simulink model "BLDC_model"  (R2021a)
settings: Solver=ode23t  StartTime=0.0  StopTime=3  RelTol=1e-3
libraries: spsMosfetLib x6, spsVoltageMeasurementLib x3, spsControlledVoltageSourceLib x1, spspowerguiLib x1
settings Model: Creator=Deepak  LastModifiedBy=Hossam
settings SolverCC: AlgebraicLoopSolver=TrustRegion
settings OptimizationCC: UseDivisionForNetSlopeComputation=on
settings DebuggingCC: SFMachineParentedDataDiag=warning
settings SFSimCC: CustomCodeUndefinedFunction=UseInterfaceOnly

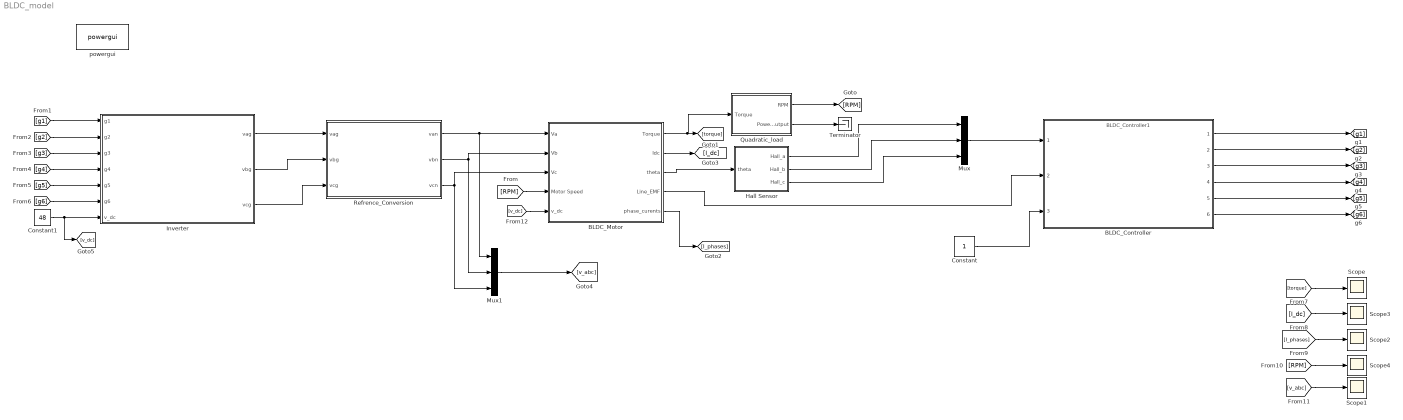
== system BLDC_model ==
  BLDC_Controller : ModelReference  ModelNameDialog=BLDC_Controller1  SimulationMode=Software-in-the-loop (SIL)  ModelReferenceVersion=2.12
  BLDC_Motor : Subsystem
  Constant : Constant  OutDataTypeStr=boolean
  Constant1 : Constant  Value=48
  Hall Sensor : Subsystem
  Inverter : Subsystem
  Mux : Mux  Inputs=3
  Mux1 : Mux  Inputs=3
  Quadratic_load : Subsystem
  Refrence_Conversion : Subsystem
  Scope{,1..4} (5 alike) : Scope
  Terminator : Terminator
  powergui : spspowerguiLib/powergui  Priority=1  SimulationMode=Discrete  SampleTime=50e-6  frequency=60  Iterations=50  frequencyindice=0  Pbase=100e6  ErrMax=1e-4  UnitsV=kV  UnitsW=MW  buscounter=0  FunctionMessages=off  echomessages=off  EnableUseOfTLC=off  CurrentSourceSwitches=off  DisableSnubberDevices=off  DisableRonSwitches=off  DisableVfSwitches=off  DisplayEquations=off  AutomaticDiscreteSolvers=off  SolverType=Tustin/Backward Euler (TBE)  Interpol=off  ExternalGateDelay=off  methode=off  Ts=100  x0status=blocks  SPID=on  SwTol=0  HookPort=off  NonlinearTolerance=0  nMaxIteration=15  ContinueOnMaxIteration=off  RestoreLinks=warning  ResistiveCurrentMeasurement=off  Frange=[0:2:500]  Ylog=off  Xlog=on  ShowGrid=off  save=off  variable=ZData  structure=0  ZoomFFT=off  StartTime=0.0  cycles=1  DisplayStyle=1  fundamental=60  FreqAxis=off  MaxFrequency=1000  frequencyindicesteady=1  RmsSteady=1  display=off
  wires:
  BLDC_Motor/3(theta) -> Hall Sensor/1(theta)
  Hall Sensor/1(Hall_a) -> Mux/1
  Hall Sensor/2(Hall_b) -> Mux/2
  Hall Sensor/3(Hall_c) -> Mux/3
  BLDC_Motor/1(Torque) -> Quadratic_load/1(Torque), [torque]
  Refrence_Conversion/2(vbn) -> Mux1/2, BLDC_Motor/2(Vb)
  Refrence_Conversion/3(vcn) -> BLDC_Motor/3(Vc), Mux1/3
  [RPM] -> BLDC_Motor/4(Motor Speed)
  Quadratic_load/1(RPM) -> [RPM]
  BLDC_Controller/1 -> [g1]
  BLDC_Controller/2 -> [g2]
  BLDC_Controller/3 -> [g3]
  BLDC_Controller/4 -> [g4]
  BLDC_Controller/5 -> [g5]
  BLDC_Controller/6 -> [g6]
  [g1] -> Inverter/1(g1)
  [g2] -> Inverter/2(g2)
  [g3] -> Inverter/3(g3)
  [g4] -> Inverter/4(g4)
  [g5] -> Inverter/5(g5)
  [g6] -> Inverter/6(g6)
  Inverter/3(vcg) -> Refrence_Conversion/3(vcg)
  Inverter/2(vbg) -> Refrence_Conversion/2(vbg)
  Inverter/1(vag) -> Refrence_Conversion/1(vag)
  Mux/1 -> BLDC_Controller/1
  Quadratic_load/2(PowerOutput) -> Terminator/1
  BLDC_Motor/2(Idc) -> [I_dc]
  Constant/1 -> BLDC_Controller/3
  BLDC_Motor/4(Line_EMF) -> BLDC_Controller/2
  [torque] -> Scope/1
  BLDC_Motor/5(phase_curents) -> [I_phases]
  [I_dc] -> Scope3/1
  [I_phases] -> Scope2/1
  [RPM] -> Scope4/1
  Mux1/1 -> [v_abc]
  [v_abc] -> Scope1/1
  Refrence_Conversion/1(van) -> Mux1/1, BLDC_Motor/1(Va)
  Constant1/1 -> [v_dc], Inverter/7(v_dc)
  [v_dc] -> BLDC_Motor/5(v_dc)

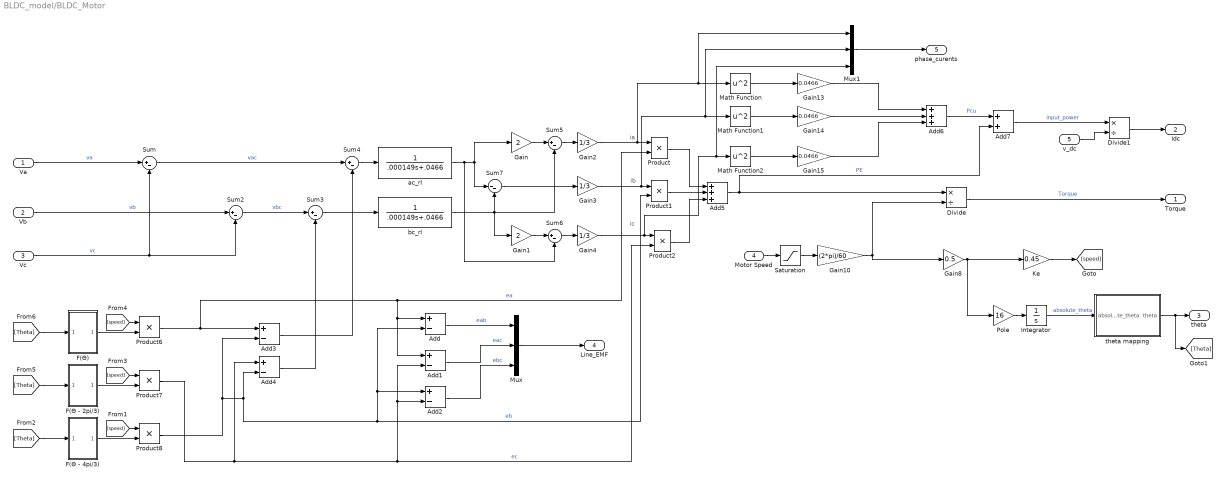
== system BLDC_model/BLDC_Motor ==
  note: ic
  note: ib
  note: ia
  Va : Inport
  Vb : Inport  Port=2
  Vc : Inport  Port=3
  Motor Speed : Inport  Port=4
  v_dc : Inport  Port=5
  Add{,2..4} (4 alike) : Sum  Inputs=+-
  Add1 : Sum  Inputs=+-  AccumDataTypeStr=double
  Add5 : Sum  Inputs=+++
  Add6 : Sum  Inputs=+++
  Add7 : Sum
  Divide : Product  Inputs=*/
  Divide1 : Product  Inputs=*/
  F(Θ - 2pi/3) : Subsystem
  F(Θ - 4pi/3) : Subsystem
  F(Θ) : Subsystem
  Gain : Gain  Gain=2
  Gain1 : Gain  Gain=2
  Gain10 : Gain  Gain=(2*pi)/60
  Gain13 : Gain  Gain=0.0466
  Gain14 : Gain  Gain=0.0466
  Gain15 : Gain  Gain=0.0466
  Gain2 : Gain  Gain=1/3
  Gain3 : Gain  Gain=1/3
  Gain4 : Gain  Gain=1/3
  Gain8 : Gain  Gain=0.5
  Integrator : Integrator
  Ke : Gain  Gain=0.45
  Math Function : Math  Operator=square  SaturateOnIntegerOverflow=on
  Math Function1 : Math  Operator=square  SaturateOnIntegerOverflow=on
  Math Function2 : Math  Operator=square  SaturateOnIntegerOverflow=on
  Mux : Mux  Inputs=3
  Mux1 : Mux  Inputs=3
  Pole : Gain  Gain=16
  Product{,1..2,6..8} (6 alike) : Product
  Saturation : Saturate  UpperLimit=50000  LowerLimit=1
  Sum{,2..6} (6 alike) : Sum  Inputs=|+-
  Sum7 : Sum  Inputs=|--
  ac_rl : TransferFcn  Denominator=[.000149 .0466]
  bc_rl : TransferFcn  Denominator=[.000149 .0466]
  theta mapping : Subsystem
  Torque : Outport
  Idc : Outport  Port=2
  theta : Outport  Port=3
  Line_EMF : Outport  Port=4
  phase_curents : Outport  Port=5
  wires:
  Pole/1 -> Integrator/1
  Sum7/1 -> Gain3/1
  Sum4/1 -> ac_rl/1
  Sum6/1 -> Gain4/1
  Add4/1 -> Sum3/2
  Vc/1 -> Sum2/2, Sum/2  "vc"
  Gain4/1 -> Mux1/3, Math Function2/1, Product2/1
  Gain2/1 -> Mux1/1, Math Function/1, Product/1
  Gain/1 -> Sum5/1
  Sum3/1 -> bc_rl/1
  Add5/1 -> Add7/2, Divide/1  "PE"
  Vb/1 -> Sum2/1  "vb"
  Sum/1 -> Sum4/1  "vac"
  bc_rl/1 -> Gain1/1, Sum5/2, Sum7/2
  Gain8/1 -> Ke/1, Pole/1
  Gain1/1 -> Sum6/1
  Product/1 -> Add5/1
  Gain3/1 -> Mux1/2, Math Function1/1, Product1/1
  Add3/1 -> Sum4/2
  Product7/1 -> Add4/1, Product2/2, Add2/2, Add1/2  "ec"
  Sum5/1 -> Gain2/1
  Product2/1 -> Add5/3
  Sum2/1 -> Sum3/1  "vbc"
  Product6/1 -> Add3/1, Add1/1, Add/1, Product/2  "ea"
  Integrator/1 -> theta mapping/1(absolute_theta)  "absolute_theta"
  Product1/1 -> Add5/2
  ac_rl/1 -> Gain/1, Sum7/1, Sum6/2
  Va/1 -> Sum/1  "va"
  Divide/1 -> Torque/1  "Torque"
  Motor Speed/1 -> Saturation/1
  Saturation/1 -> Gain10/1
  Math Function/1 -> Gain13/1
  Math Function1/1 -> Gain14/1
  Math Function2/1 -> Gain15/1
  Gain13/1 -> Add6/1
  Gain14/1 -> Add6/2
  Gain15/1 -> Add6/3
  Add6/1 -> Add7/1  "Pcu"
  Add7/1 -> Divide1/1  "input_power"
  Divide1/1 -> Idc/1
  Add/1 -> Mux/1  "eab"
  Add1/1 -> Mux/2  "eac"
  Add2/1 -> Mux/3  "ebc"
  Mux/1 -> Line_EMF/1
  Gain10/1 -> Divide/2, Gain8/1
  Ke/1 -> [speed]
  theta mapping/1(theta) -> [Theta], theta/1
  F(Θ)/1(Out1) -> Product6/2
  F(Θ - 2pi/3)/1(Out1) -> Product7/2
  F(Θ - 4pi/3)/1(Out1) -> Product8/2
  Product8/1 -> Add3/2, Product1/2, Add/2, Add2/1, Add4/2  "eb"
  [speed] -> Product8/1
  [speed] -> Product7/1
  [speed] -> Product6/1
  [Theta] -> F(Θ - 4pi/3)/1(In1)
  [Theta] -> F(Θ - 2pi/3)/1(In1)
  [Theta] -> F(Θ)/1(In1)
  Mux1/1 -> phase_curents/1
  v_dc/1 -> Divide1/2

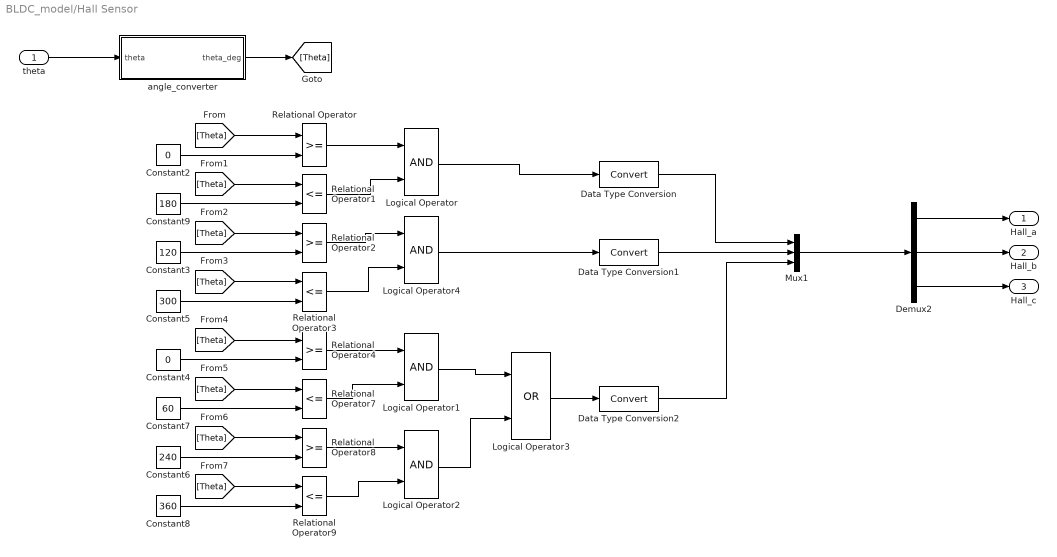
== system BLDC_model/Hall Sensor ==
  theta : Inport
  Constant2 : Constant  Value=0
  Constant3 : Constant  Value=120
  Constant4 : Constant  Value=0
  Constant5 : Constant  Value=300
  Constant6 : Constant  Value=240
  Constant7 : Constant  Value=60
  Constant8 : Constant  Value=360
  Constant9 : Constant  Value=180
  Data Type Conversion : DataTypeConversion
  Data Type Conversion1 : DataTypeConversion
  Data Type Conversion2 : DataTypeConversion
  Demux2 : Demux  Outputs=3
  Logical Operator{,1..2,4} (4 alike) : Logic  AllPortsSameDT=off  OutDataTypeStr=boolean
  Logical Operator3 : Logic  Operator=OR  AllPortsSameDT=off  OutDataTypeStr=boolean
  Mux1 : Mux  Inputs=3
  Relational Operator{,2,4,8} (4 alike) : RelationalOperator  OutDataTypeStr=boolean  RndMeth=Nearest
  Relational Operator{1,3,7,9} (4 alike) : RelationalOperator  Operator=<=  OutDataTypeStr=boolean  RndMeth=Nearest
  angle_converter : Subsystem
  Hall_a : Outport
  Hall_b : Outport  Port=2
  Hall_c : Outport  Port=3
  wires:
  Constant7/1 -> Relational Operator7/2
  Constant3/1 -> Relational Operator2/2
  Relational Operator1/1 -> Logical Operator/2
  Constant9/1 -> Relational Operator1/2
  Relational Operator7/1 -> Logical Operator1/2
  Relational Operator4/1 -> Logical Operator1/1
  Constant2/1 -> Relational Operator/2
  Data Type Conversion/1 -> Mux1/1
  Mux1/1 -> Demux2/1
  Constant4/1 -> Relational Operator4/2
  Relational Operator2/1 -> Logical Operator4/1
  Data Type Conversion1/1 -> Mux1/2
  Constant5/1 -> Relational Operator3/2
  theta/1 -> angle_converter/1(theta)
  Relational Operator/1 -> Logical Operator/1
  Relational Operator3/1 -> Logical Operator4/2
  Logical Operator4/1 -> Data Type Conversion1/1
  Data Type Conversion2/1 -> Mux1/3
  Logical Operator/1 -> Data Type Conversion/1
  Demux2/2 -> Hall_b/1
  Relational Operator8/1 -> Logical Operator2/1
  Relational Operator9/1 -> Logical Operator2/2
  Constant6/1 -> Relational Operator8/2
  Logical Operator1/1 -> Logical Operator3/1
  Logical Operator2/1 -> Logical Operator3/2
  Logical Operator3/1 -> Data Type Conversion2/1
  Demux2/3 -> Hall_c/1
  Demux2/1 -> Hall_a/1
  angle_converter/1(theta_deg) -> [Theta]
  [Theta] -> Relational Operator/1
  [Theta] -> Relational Operator1/1
  [Theta] -> Relational Operator2/1
  [Theta] -> Relational Operator3/1
  [Theta] -> Relational Operator4/1
  [Theta] -> Relational Operator7/1
  [Theta] -> Relational Operator8/1
  Constant8/1 -> Relational Operator9/2
  [Theta] -> Relational Operator9/1

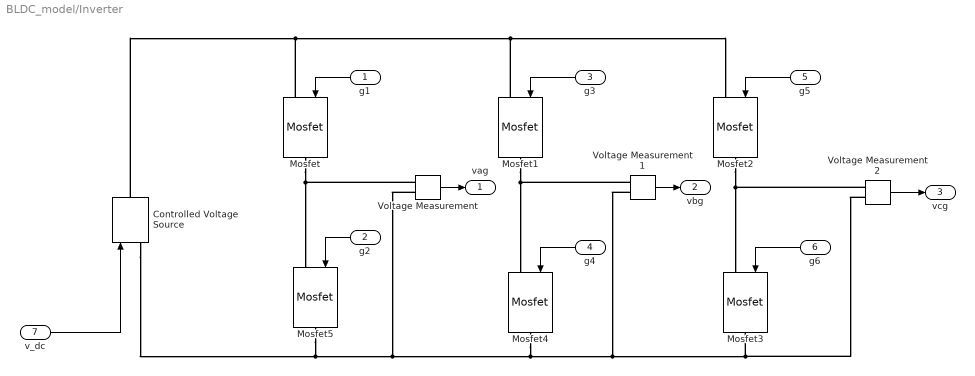
== system BLDC_model/Inverter ==
  g1 : Inport
  g2 : Inport  Port=2
  g3 : Inport  Port=3
  g4 : Inport  Port=4
  g5 : Inport  Port=5
  g6 : Inport  Port=6
  v_dc : Inport  Port=7
  Controlled Voltage Source : spsControlledVoltageSourceLib/Controlled Voltage Source  Initialize=on  Source_Type=DC  Amplitude=48  Phase=0  Frequency=0  Measurements=None
  Mosfet{,1..5} (6 alike) : spsMosfetLib/Mosfet  Ron=0.1  Lon=0  Rd=0.01  Vfd=0  IC=0  Rs=1e5  Cs=inf  Measurements=off
  Voltage Measurement : spsVoltageMeasurementLib/Voltage Measurement  PhasorSimulation=off  OutputType=Complex  PSBequivalent=0
  Voltage Measurement1 : spsVoltageMeasurementLib/Voltage Measurement  PhasorSimulation=off  OutputType=Complex  PSBequivalent=0
  Voltage Measurement2 : spsVoltageMeasurementLib/Voltage Measurement  PhasorSimulation=off  OutputType=Complex  PSBequivalent=0
  vag : Outport
  vbg : Outport  Port=2
  vcg : Outport  Port=3
  wires:
  v_dc/1 -> Controlled Voltage Source/1
  g6/1 -> Mosfet3/1
  g4/1 -> Mosfet4/1
  g3/1 -> Mosfet1/1
  g1/1 -> Mosfet/1
  g5/1 -> Mosfet2/1
  g2/1 -> Mosfet5/1
  Voltage Measurement/1 -> vag/1
  Voltage Measurement1/1 -> vbg/1
  Voltage Measurement2/1 -> vcg/1
  connections:
  Mosfet/LConn1 -- Controlled Voltage Source/RConn1 -- Mosfet1/LConn1 -- Mosfet2/LConn1
  Mosfet2/RConn1 -- Voltage Measurement2/LConn1 -- Mosfet3/LConn1
  Mosfet5/RConn1 -- Mosfet4/RConn1 -- Mosfet3/RConn1 -- Voltage Measurement2/LConn2 -- Voltage Measurement1/LConn2 -- Voltage Measurement/LConn2 -- Controlled Voltage Source/LConn1
  Mosfet1/RConn1 -- Mosfet4/LConn1 -- Voltage Measurement1/LConn1
  Mosfet/RConn1 -- Voltage Measurement/LConn1 -- Mosfet5/LConn1

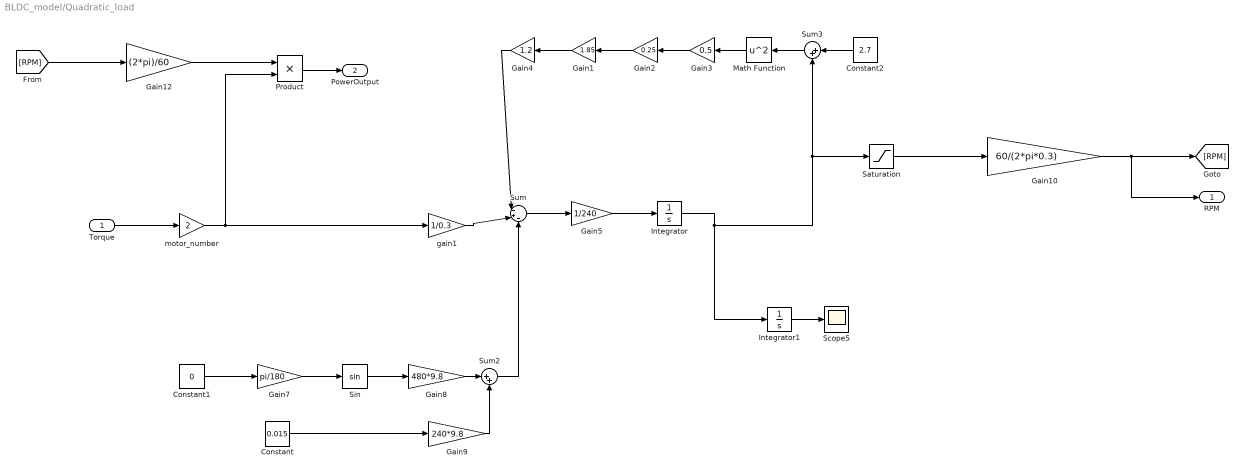
== system BLDC_model/Quadratic_load ==
  Torque : Inport
  Constant : Constant  Value=0.015
  Constant1 : Constant  Value=0
  Constant2 : Constant  Value=2.7
  Gain1 : Gain  Gain=1.85
  Gain10 : Gain  Gain=60/(2*pi*0.3)
  Gain12 : Gain  Gain=(2*pi)/60
  Gain2 : Gain  Gain=0.25
  Gain3 : Gain  Gain=0.5
  Gain4 : Gain  Gain=1.2
  Gain5 : Gain  Gain=1/240
  Gain7 : Gain  Gain=pi/180
  Gain8 : Gain  Gain=480*9.8
  Gain9 : Gain  Gain=240*9.8
  Integrator : Integrator
  Integrator1 : Integrator
  Math Function : Math  Operator=square  SaturateOnIntegerOverflow=on
  Product : Product
  Saturation : Saturate  UpperLimit=50000  LowerLimit=0
  Scope5 : Scope
  Sin : Trigonometry
  Sum : Sum  Inputs=|-+-
  Sum2 : Sum  Inputs=|++
  Sum3 : Sum  Inputs=|++
  gain1 : Gain  Gain=1/0.3
  motor_number : Gain  Gain=2
  RPM : Outport
  PowerOutput : Outport  Port=2
  wires:
  Gain10/1 -> RPM/1, [RPM]
  Sum2/1 -> Sum/3
  Gain7/1 -> Sin/1
  Gain8/1 -> Sum2/1
  Sin/1 -> Gain8/1
  Gain9/1 -> Sum2/2
  Gain2/1 -> Gain1/1
  Gain4/1 -> Sum/1
  gain1/1 -> Sum/2
  Gain1/1 -> Gain4/1
  Sum3/1 -> Math Function/1
  Constant2/1 -> Sum3/1
  Integrator/1 -> Integrator1/1, Saturation/1, Sum3/2
  Product/1 -> PowerOutput/1
  Gain5/1 -> Integrator/1
  Constant1/1 -> Gain7/1
  Constant/1 -> Gain9/1
  Sum/1 -> Gain5/1
  Math Function/1 -> Gain3/1
  Gain3/1 -> Gain2/1
  Torque/1 -> motor_number/1
  Saturation/1 -> Gain10/1
  motor_number/1 -> Product/2, gain1/1
  Integrator1/1 -> Scope5/1
  [RPM] -> Gain12/1
  Gain12/1 -> Product/1

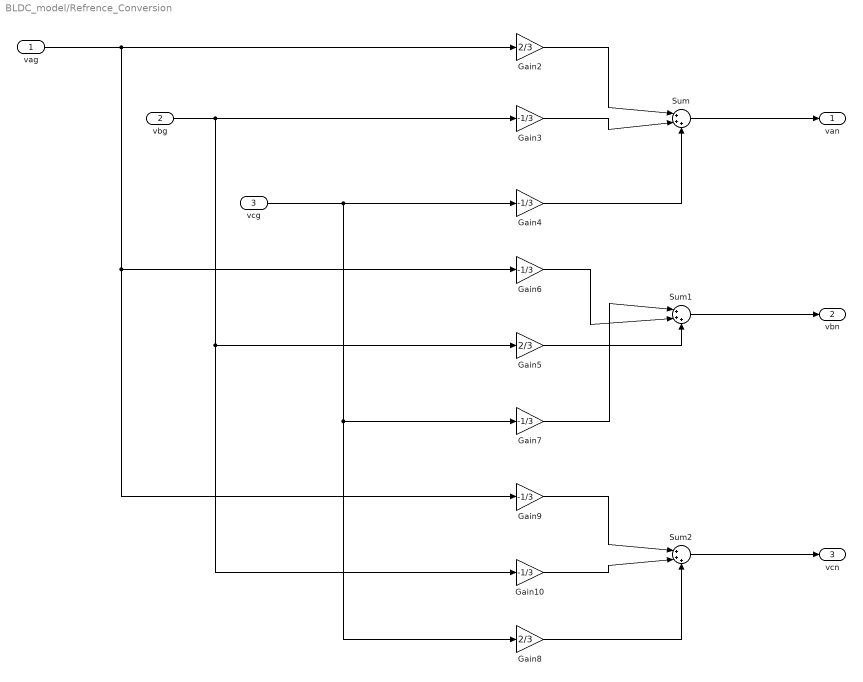
== system BLDC_model/Refrence_Conversion ==
  vag : Inport
  vbg : Inport  Port=2
  vcg : Inport  Port=3
  Gain{3..4,6..7,9..10} (6 alike) : Gain  Gain=-1/3
  Gain2 : Gain  Gain=2/3
  Gain5 : Gain  Gain=2/3
  Gain8 : Gain  Gain=2/3
  Sum : Sum  Inputs=|+++
  Sum1 : Sum  Inputs=|+++
  Sum2 : Sum  Inputs=|+++
  van : Outport
  vbn : Outport  Port=2
  vcn : Outport  Port=3
  wires:
  Gain10/1 -> Sum2/2
  Gain9/1 -> Sum2/1
  Gain8/1 -> Sum2/3
  Gain7/1 -> Sum1/1
  Gain4/1 -> Sum/3
  Gain3/1 -> Sum/2
  vbg/1 -> Gain10/1, Gain5/1, Gain3/1
  Gain6/1 -> Sum1/2
  Gain2/1 -> Sum/1
  vcg/1 -> Gain8/1, Gain7/1, Gain4/1
  Gain5/1 -> Sum1/3
  vag/1 -> Gain2/1, Gain6/1, Gain9/1
  Sum/1 -> van/1
  Sum1/1 -> vbn/1
  Sum2/1 -> vcn/1

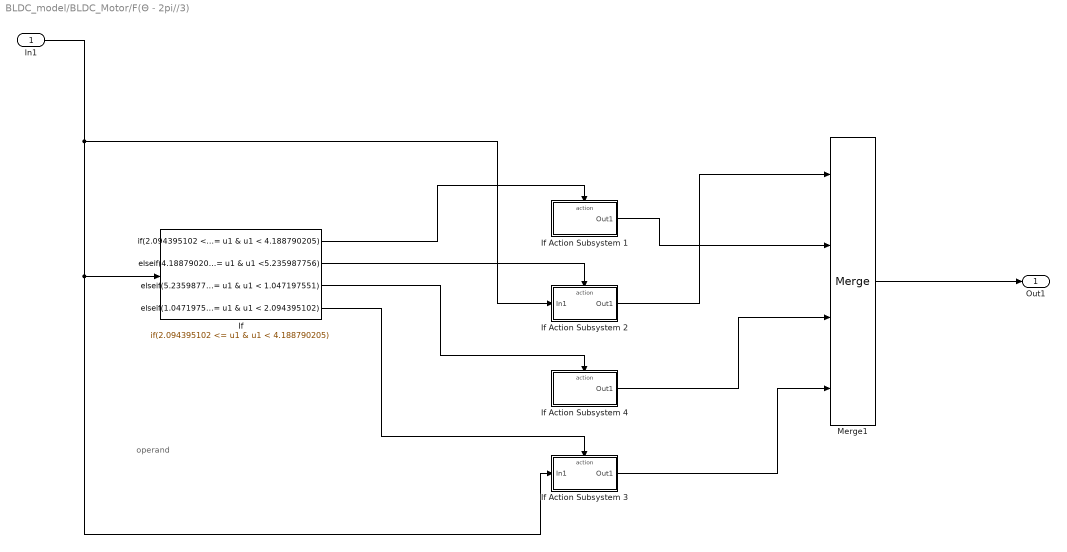
== system BLDC_model/BLDC_Motor/F(Θ - 2pi//3) ==
  note: operand
  In1 : Inport
  If : If  IfExpression=2.094395102 <= u1 & u1 < 4.188790205  ElseIfExpressions=4.188790205 <= u1 & u1 <5.235987756 , 5.235987756>= u1 & u1 < 1.047197551 , 1.047197551 <= u1 & u1 < 2.094395102  ShowElse=off
  If Action Subsystem 1 : Subsystem  TreatAsAtomicUnit=on
  If Action Subsystem 2 : Subsystem  TreatAsAtomicUnit=on
  If Action Subsystem 3 : Subsystem  TreatAsAtomicUnit=on
  If Action Subsystem 4 : Subsystem  TreatAsAtomicUnit=on
  Merge1 : Merge  Inputs=4
  Out1 : Outport
  wires:
  If/3 -> If Action Subsystem 4/Action
  If Action Subsystem 2/1(Out1) -> Merge1/1
  If Action Subsystem 4/1(Out1) -> Merge1/3
  If/4 -> If Action Subsystem 3/Action
  If/2 -> If Action Subsystem 2/Action
  If Action Subsystem 3/1(Out1) -> Merge1/4
  If/1 -> If Action Subsystem 1/Action
  If Action Subsystem 1/1(Out1) -> Merge1/2
  Merge1/1 -> Out1/1
  In1/1 -> If Action Subsystem 3/1(In1), If/1, If Action Subsystem 2/1(In1)

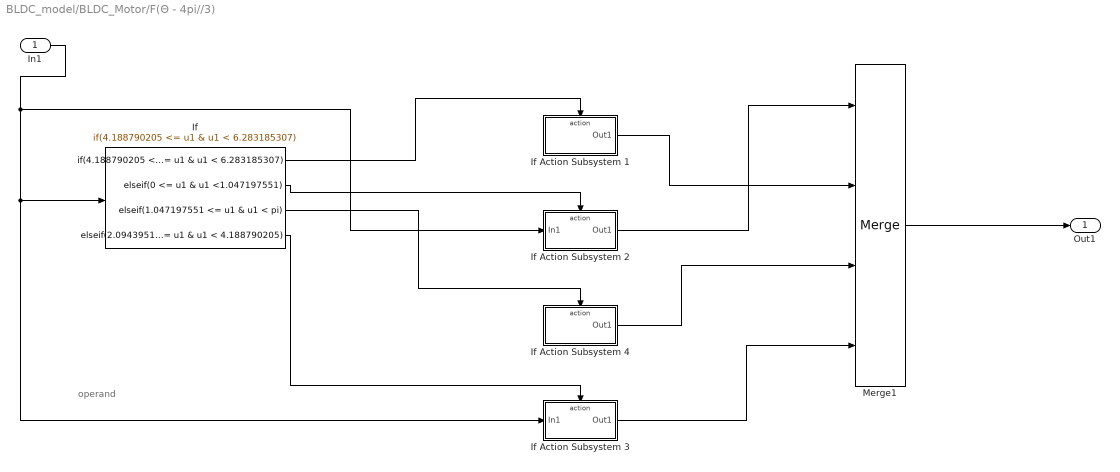
== system BLDC_model/BLDC_Motor/F(Θ - 4pi//3) ==
  note: operand
  In1 : Inport
  If : If  IfExpression=4.188790205 <= u1 & u1 < 6.283185307  ElseIfExpressions=0 <= u1 & u1 <1.047197551 , 1.047197551 <= u1 & u1 < pi , 2.094395102 <= u1 & u1 < 4.188790205  ShowElse=off
  If Action Subsystem 1 : Subsystem  TreatAsAtomicUnit=on
  If Action Subsystem 2 : Subsystem  TreatAsAtomicUnit=on
  If Action Subsystem 3 : Subsystem  TreatAsAtomicUnit=on
  If Action Subsystem 4 : Subsystem  TreatAsAtomicUnit=on
  Merge1 : Merge  Inputs=4
  Out1 : Outport
  wires:
  If/3 -> If Action Subsystem 4/Action
  If Action Subsystem 2/1(Out1) -> Merge1/1
  If Action Subsystem 4/1(Out1) -> Merge1/3
  If/4 -> If Action Subsystem 3/Action
  If/2 -> If Action Subsystem 2/Action
  If Action Subsystem 3/1(Out1) -> Merge1/4
  If/1 -> If Action Subsystem 1/Action
  If Action Subsystem 1/1(Out1) -> Merge1/2
  Merge1/1 -> Out1/1
  In1/1 -> If Action Subsystem 2/1(In1), If Action Subsystem 3/1(In1), If/1

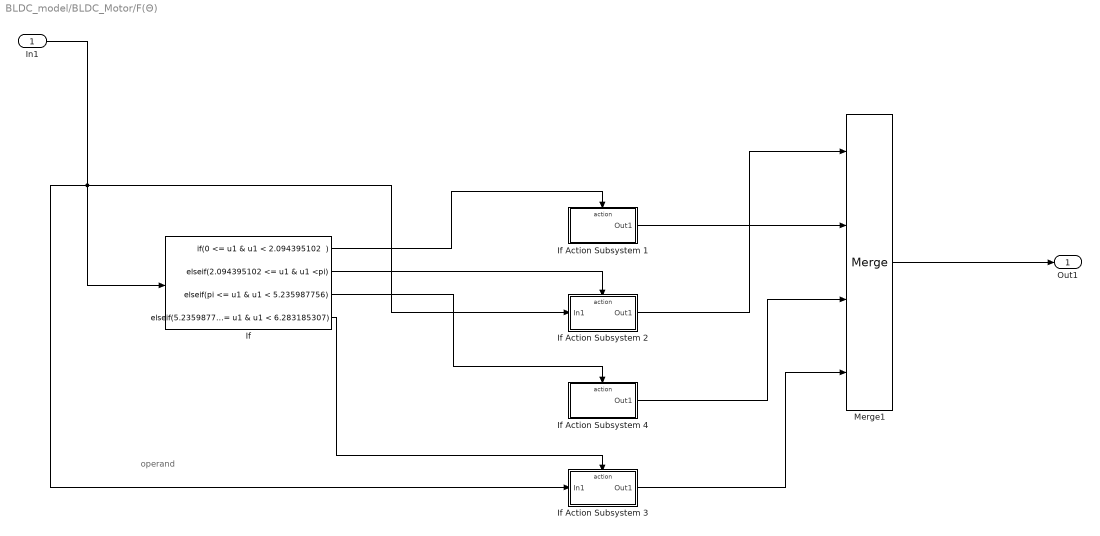
== system BLDC_model/BLDC_Motor/F(Θ) ==
  note: operand
  In1 : Inport
  If : If  IfExpression=0 <= u1 & u1 < 2.094395102  ElseIfExpressions=2.094395102 <= u1 & u1 <pi , pi <= u1 & u1 < 5.235987756 , 5.235987756 <= u1 & u1 < 6.283185307  ShowElse=off
  If Action Subsystem 1 : Subsystem  TreatAsAtomicUnit=on
  If Action Subsystem 2 : Subsystem  TreatAsAtomicUnit=on
  If Action Subsystem 3 : Subsystem  TreatAsAtomicUnit=on
  If Action Subsystem 4 : Subsystem  TreatAsAtomicUnit=on
  Merge1 : Merge  Inputs=4
  Out1 : Outport
  wires:
  If/3 -> If Action Subsystem 4/Action
  If Action Subsystem 2/1(Out1) -> Merge1/1
  If Action Subsystem 4/1(Out1) -> Merge1/3
  If/4 -> If Action Subsystem 3/Action
  If/2 -> If Action Subsystem 2/Action
  If Action Subsystem 3/1(Out1) -> Merge1/4
  If/1 -> If Action Subsystem 1/Action
  If Action Subsystem 1/1(Out1) -> Merge1/2
  Merge1/1 -> Out1/1
  In1/1 -> If Action Subsystem 2/1(In1), If Action Subsystem 3/1(In1), If/1

== system BLDC_model/BLDC_Motor/theta mapping ==
  absolute_theta : Inport
  If : If  IfExpression=u1 >= 6.283185307
  If Action Subsystem 1 : Subsystem  TreatAsAtomicUnit=on
  If Action Subsystem 2 : Subsystem  TreatAsAtomicUnit=on
  Merge1 : Merge
  theta : Outport
  wires:
  absolute_theta/1 -> If Action Subsystem 2/1(In1), If Action Subsystem 1/1(In1), If/1
  If Action Subsystem 1/1(Out1) -> Merge1/1
  If/1 -> If Action Subsystem 1/Action
  If/2 -> If Action Subsystem 2/Action
  If Action Subsystem 2/1(Out1) -> Merge1/2
  Merge1/1 -> theta/1

== system BLDC_model/Hall Sensor/angle_converter ==
  theta : Inport
  rad2deg : Gain  Gain=180/pi
  theta_deg : Outport
  wires:
  rad2deg/1 -> theta_deg/1
  theta/1 -> rad2deg/1

== system BLDC_model/BLDC_Motor/F(Θ - 2pi//3)/If Action Subsystem 1 ==
  Action Port : ActionPort  ActionPortLabel=if(2.094395102 <= u1 & u1 < 4.188790205)
  Constant : Constant
  Out1 : Outport  VectorParamsAs1DForOutWhenUnconnected=off
  wires:
  Constant/1 -> Out1/1

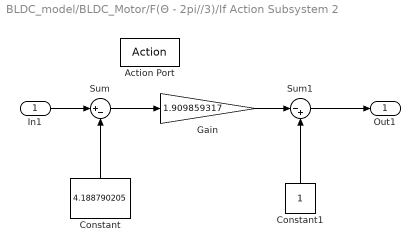
== system BLDC_model/BLDC_Motor/F(Θ - 2pi//3)/If Action Subsystem 2 ==
  In1 : Inport
  Action Port : ActionPort  ActionPortLabel=elseif(4.188790205 <= u1 & u1 <5.235987756 )
  Constant : Constant  Value=4.188790205
  Constant1 : Constant
  Gain : Gain  Gain=1.909859317
  Sum : Sum  Inputs=|+-
  Sum1 : Sum  Inputs=|-+
  Out1 : Outport  VectorParamsAs1DForOutWhenUnconnected=off
  wires:
  In1/1 -> Sum/1
  Constant/1 -> Sum/2
  Sum/1 -> Gain/1
  Constant1/1 -> Sum1/2
  Gain/1 -> Sum1/1
  Sum1/1 -> Out1/1

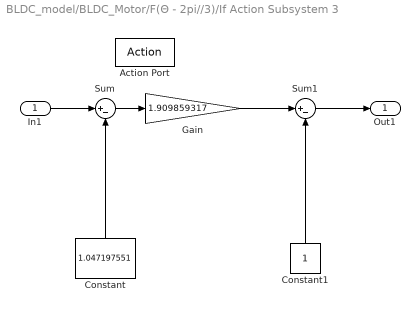
== system BLDC_model/BLDC_Motor/F(Θ - 2pi//3)/If Action Subsystem 3 ==
  In1 : Inport
  Action Port : ActionPort  ActionPortLabel=elseif( 1.047197551 <= u1 & u1 < 2.094395102)
  Constant : Constant  Value=1.047197551
  Constant1 : Constant
  Gain : Gain  Gain=1.909859317
  Sum : Sum  Inputs=|+-
  Sum1 : Sum  Inputs=|+-
  Out1 : Outport  VectorParamsAs1DForOutWhenUnconnected=off
  wires:
  Constant1/1 -> Sum1/2
  Sum/1 -> Gain/1
  Gain/1 -> Sum1/1
  In1/1 -> Sum/1
  Constant/1 -> Sum/2
  Sum1/1 -> Out1/1

== system BLDC_model/BLDC_Motor/F(Θ - 2pi//3)/If Action Subsystem 4 ==
  Action Port : ActionPort  ActionPortLabel=elseif( 5.235987756>= u1 & u1 < 1.047197551 )
  Constant : Constant  Value=-1
  Out1 : Outport  VectorParamsAs1DForOutWhenUnconnected=off
  wires:
  Constant/1 -> Out1/1

== system BLDC_model/BLDC_Motor/F(Θ - 4pi//3)/If Action Subsystem 1 ==
  Action Port : ActionPort  ActionPortLabel=if(4.188790205 <= u1 & u1 < 6.283185307)
  Constant : Constant
  Out1 : Outport  VectorParamsAs1DForOutWhenUnconnected=off
  wires:
  Constant/1 -> Out1/1

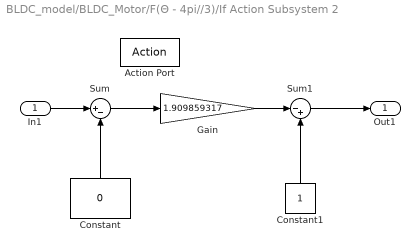
== system BLDC_model/BLDC_Motor/F(Θ - 4pi//3)/If Action Subsystem 2 ==
  In1 : Inport
  Action Port : ActionPort  ActionPortLabel=elseif(0 <= u1 & u1 <1.047197551 )
  Constant : Constant  Value=0
  Constant1 : Constant
  Gain : Gain  Gain=1.909859317
  Sum : Sum  Inputs=|+-
  Sum1 : Sum  Inputs=|-+
  Out1 : Outport  VectorParamsAs1DForOutWhenUnconnected=off
  wires:
  In1/1 -> Sum/1
  Constant/1 -> Sum/2
  Sum/1 -> Gain/1
  Constant1/1 -> Sum1/2
  Gain/1 -> Sum1/1
  Sum1/1 -> Out1/1

== system BLDC_model/BLDC_Motor/F(Θ - 4pi//3)/If Action Subsystem 3 ==
  In1 : Inport
  Action Port : ActionPort  ActionPortLabel=elseif( 2.094395102 <= u1 & u1 < 4.188790205)
  Constant : Constant  Value=pi
  Constant1 : Constant
  Gain : Gain  Gain=1.909859317
  Sum : Sum  Inputs=|+-
  Sum1 : Sum  Inputs=|+-
  Out1 : Outport  VectorParamsAs1DForOutWhenUnconnected=off
  wires:
  Constant1/1 -> Sum1/2
  Sum/1 -> Gain/1
  Gain/1 -> Sum1/1
  In1/1 -> Sum/1
  Constant/1 -> Sum/2
  Sum1/1 -> Out1/1

== system BLDC_model/BLDC_Motor/F(Θ - 4pi//3)/If Action Subsystem 4 ==
  Action Port : ActionPort  ActionPortLabel=elseif( 1.047197551 <= u1 & u1 < pi )
  Constant : Constant  Value=-1
  Out1 : Outport  VectorParamsAs1DForOutWhenUnconnected=off
  wires:
  Constant/1 -> Out1/1

== system BLDC_model/BLDC_Motor/F(Θ)/If Action Subsystem 1 ==
  Action Port : ActionPort  ActionPortLabel="if(0 <= u1 & u1 < 2.094395102  )"
  Constant : Constant
  Out1 : Outport  VectorParamsAs1DForOutWhenUnconnected=off
  wires:
  Constant/1 -> Out1/1

== system BLDC_model/BLDC_Motor/F(Θ)/If Action Subsystem 2 ==
  In1 : Inport
  Action Port : ActionPort  ActionPortLabel=elseif(2.094395102 <= u1 & u1 <pi )
  Constant : Constant  Value=2.094395102
  Constant1 : Constant
  Gain : Gain  Gain=1.909859317
  Sum : Sum  Inputs=|+-
  Sum1 : Sum  Inputs=|-+
  Out1 : Outport  VectorParamsAs1DForOutWhenUnconnected=off
  wires:
  In1/1 -> Sum/1
  Constant/1 -> Sum/2
  Sum/1 -> Gain/1
  Constant1/1 -> Sum1/2
  Gain/1 -> Sum1/1
  Sum1/1 -> Out1/1

== system BLDC_model/BLDC_Motor/F(Θ)/If Action Subsystem 3 ==
  In1 : Inport
  Action Port : ActionPort  ActionPortLabel=elseif( 5.235987756 <= u1 & u1 < 6.283185307)
  Constant : Constant  Value=5.235987756
  Constant1 : Constant
  Gain : Gain  Gain=1.909859317
  Sum : Sum  Inputs=|+-
  Sum1 : Sum  Inputs=|+-
  Out1 : Outport  VectorParamsAs1DForOutWhenUnconnected=off
  wires:
  Constant1/1 -> Sum1/2
  Sum/1 -> Gain/1
  Gain/1 -> Sum1/1
  In1/1 -> Sum/1
  Constant/1 -> Sum/2
  Sum1/1 -> Out1/1

== system BLDC_model/BLDC_Motor/F(Θ)/If Action Subsystem 4 ==
  Action Port : ActionPort  ActionPortLabel=elseif( pi <= u1 & u1 < 5.235987756 )
  Constant : Constant  Value=-1
  Out1 : Outport  VectorParamsAs1DForOutWhenUnconnected=off
  wires:
  Constant/1 -> Out1/1

== system BLDC_model/BLDC_Motor/theta mapping/If Action Subsystem 1 ==
  In1 : Inport
  Action Port : ActionPort  ActionPortLabel=if(u1 >= 6.283185307)
  Constant : Constant  Value=6.283185307
  Divide : Product  Inputs=*/
  Floor : Rounding
  Product : Product
  Sum : Sum  Inputs=|+-
  Out1 : Outport  VectorParamsAs1DForOutWhenUnconnected=off
  wires:
  In1/1 -> Sum/1, Divide/1
  Constant/1 -> Product/2, Divide/2
  Divide/1 -> Floor/1
  Floor/1 -> Product/1
  Product/1 -> Sum/2
  Sum/1 -> Out1/1

== system BLDC_model/BLDC_Motor/theta mapping/If Action Subsystem 2 ==
  In1 : Inport
  Action Port : ActionPort  ActionPortLabel=else
  Out1 : Outport  VectorParamsAs1DForOutWhenUnconnected=off
  wires:
  In1/1 -> Out1/1
